simulink model "proj1_week1"  (R2021a)
settings: Solver=VariableStepAuto  StartTime=0.0  StopTime=10.0  RelTol=1e-3
model workspace (MAT data in the model file):
  K12 = Simulink.Parameter
  K12.Value = 4000
  K12.DataType = 'auto'
  K12.Dimensions = [1 1]
  M1 = Simulink.Parameter
  M1.Value = 100
  M1.DataType = 'auto'
  M1.Dimensions = [1 1]
  M2 = Simulink.Parameter
  M2.Value = 50
  M2.DataType = 'auto'
  M2.Dimensions = [1 1]
  b = Simulink.Parameter
  b.Value = 50
  b.DataType = 'auto'
  b.Dimensions = [1 1]
  k1 = Simulink.Parameter
  k1.Value = 50
  k1.DataType = 'auto'
  k1.Dimensions = [1 1]
settings Model: Creator=RASIKA MALGI  LastModifiedBy=RASIKA MALGI

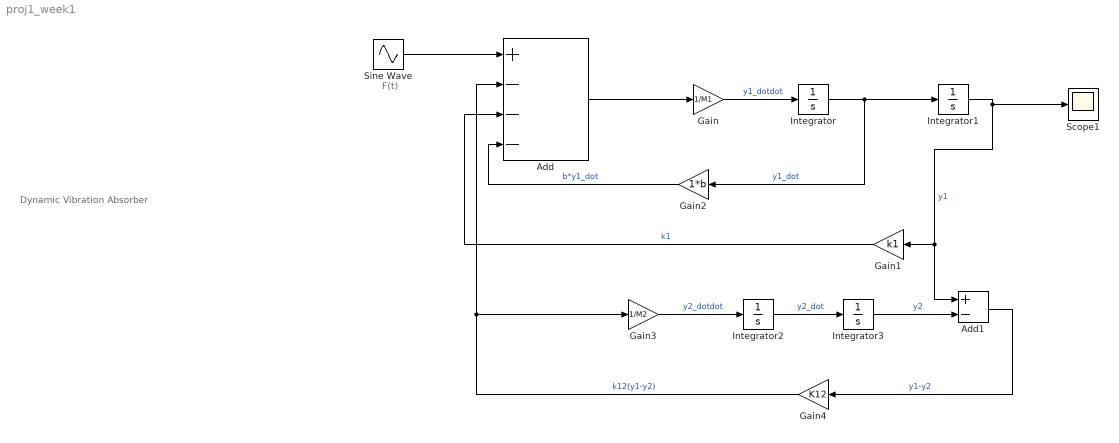
== system proj1_week1 ==
  note: Dynamic Vibration Absorber
  note: F(t)
  Add : Sum  Inputs=+---
  Add1 : Sum  Inputs=+-
  Gain : Gain  Gain=1/M1
  Gain1 : Gain  Gain=k1
  Gain2 : Gain  Gain=1*b
  Gain3 : Gain  Gain=1/M2
  Gain4 : Gain  Gain=K12
  Integrator{,1..3} (4 alike) : Integrator
  Scope1 : Scope
  Sine Wave : Sin  SampleTime=0
  wires:
  Gain2/1 -> Add/4  "b*y1_dot"
  Integrator3/1 -> Add1/2  "y2"
  Integrator2/1 -> Integrator3/1  "y2_dot"
  Gain3/1 -> Integrator2/1  "y2_dotdot"
  Add1/1 -> Gain4/1  "y1-y2"
  Gain/1 -> Integrator/1  "y1_dotdot"
  Sine Wave/1 -> Add/1
  Integrator1/1 -> Scope1/1, Gain1/1, Add1/1  "y1"
  Add/1 -> Gain/1
  Gain4/1 -> Gain3/1, Add/2  "k12(y1-y2)"
  Gain1/1 -> Add/3  "k1"
  Integrator/1 -> Gain2/1, Integrator1/1  "y1_dot"
